simulink model "TV_2018_HIL"  (R2016a)
settings: Solver=FixedStepAuto  StartTime=0.0  StopTime=inf  FixedStep=0.001  RelTol=1e-3
PreLoadFcn:
  | TV_2017_parameters
values from neighbouring files (symbols this model uses):
  battery_voltage = single(530)    [HIL_parameters.m]    (also in HIL_parameters_2018.m; TV_2017_parameters.m; TV_2017_parameters_VD.m)
  car_params = Simulink_Car_params    [HIL_parameters.m]    (also in HIL_parameters_2018.m; TV_2017_parameters.m; TV_2017_parameters_VD.m)
  i_Diff = 16    [HIL_parameters.m]    (also in HIL_parameters_2018.m; TV_2017_parameters.m)
  Kp = 1    [HIL_parameters.m]    (also in HIL_parameters_2018.m; TV_2017_parameters.m; TV_2017_parameters_VD.m)
  motor_data = struct    [HIL_parameters.m]    (also in HIL_parameters_2018.m; TV_2017_parameters.m)
  powerLimitControl = Simulink_el    [HIL_parameters.m]    (also in HIL_parameters_2018.m; TV_2017_parameters.m; TV_2017_parameters_VD.m)
  settings = Simulink_Settings    [HIL_parameters.m]    (also in HIL_parameters_2018.m; TV_2017_parameters.m; TV_2017_parameters_VD.m)
  SpdC_BCC = 0    [HIL_parameters.m]    (also in HIL_parameters_2018.m; TV_2017_parameters.m; TV_2017_parameters_VD.m)
  Speed_Neg_sat = -21    [HIL_parameters.m]    (also in HIL_parameters_2018.m; TV_2017_parameters.m; TV_2017_parameters_VD.m)
  Speed_Pos_sat = 21    [HIL_parameters.m]    (also in HIL_parameters_2018.m; TV_2017_parameters.m; TV_2017_parameters_VD.m)
  SteeringAngleFL = [-23.80 -22.65 -21.50 -20.34 -19.18 -18.03 -16.86 -15.70 -14.53 -13.35 -12.18 -10.99 -9.80 -8.61 -7.40 -6.19 -4.97 -3.75 -2.51 -1.26 0 1.27 2.56 3.85 5.17 6.50 7.84 9.21 10.59 12.00 13.42 14.88 16.36 17.87 19.41 20.99 22.61 24.26 25.97 27.73 29.54]    [CarSetupAnalysis2018.m]    (also in HIL_parameters_2018.m; TV_2017_parameters.m; TV_2017_parameters_VD.m = [-24.129 -22.950 -21.772 -20.593 -19.413 -18.232 -17.050 -15)
  SteeringAngleFR = [-29.54 -27.73 -25.97 -24.26 -22.61 -20.99 -19.41 -17.87 -16.36 -14.88 -13.42 -12.00 -10.59 -9.21 -7.84 -6.50 -5.17 -3.85 -2.56 -1.27 0 1.26 2.51 3.75 4.97 6.19 7.40 8.61 9.80 10.99 12.18 13.35 14.53 15.70 16.86 18.03 19.18 20.34 21.50 22.65 23.80]    [CarSetupAnalysis2018.m]    (also in HIL_parameters_2018.m; TV_2017_parameters.m; TV_2017_parameters_VD.m = [-29.3050 -27.5340 -25.8140 -24.1410 -22.5110 -20.9180 -19.3)
  SteeringWhAngle = [-105 -99.75 -94.5 -89.25 -84 -78.75 -73.5 -68.25 -63 -57.75 -52.5 -47.25 -42 -36.75 -31.5 -26.25 -21.0 -15.75 -10.5 -5.25 0.0 5.25 10.50 15.75 21.00 26.25 31.50 36.75 42.00 47.25 52.50 57.75  63.00 68.25 73.50 78.75 84.00 89.25 94.50 99.75 105.00]    [TV_2017_parameters_VD.m]
  Tn_n = 0    [HIL_parameters.m]    (also in HIL_parameters_2018.m; TV_2017_parameters.m; TV_2017_parameters_VD.m)
  tractionControl = Simulink_tc    [HIL_parameters.m]    (also in HIL_parameters_2018.m; IterativeTractionControlTuning.m; TV_2017_parameters.m; TV_2017_parameters_VD.m)
  yawMomentGenerator = struct    [HIL_parameters.m]    (also in HIL_parameters_2018.m = Simulink_yawRate2; TV_2017_parameters.m = Simulink_yawRate2)
  yawRateControl = Simulink_yawRate    [HIL_parameters.m]    (also in HIL_parameters_2018.m; TV_2017_parameters.m; TV_2017_parameters_VD.m)
undefined symbols (not defined in the file or in its folder): canChannel, DiscIntNeverNeededParam, magnitude, speedEstimation, TC_Decr_Gas, TC_Derivative, TC_Incr_Gas, TC_On, TC_Relay_Off, TC_Relay_On
libraries: CarMaker4SL x366, simulink_extras x63, canmsglib x55, canlib x41, simulink x37, dspfdesign x2, sldrtlib x1
(part 3 of 15)

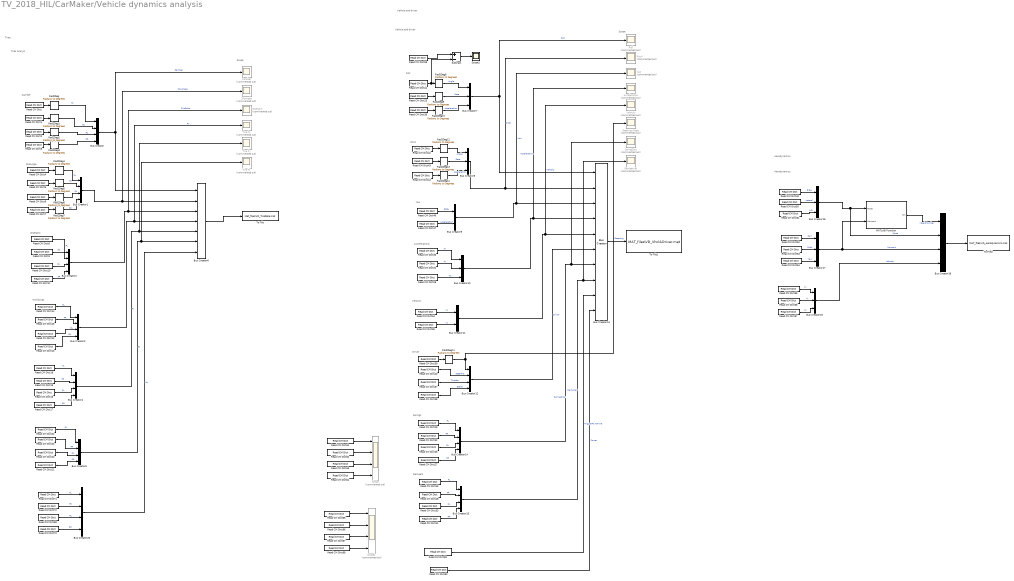
== system TV_2018_HIL/CarMaker/Vehicle dynamics analysis ==
  note: Aerodynamics
  note: Scope
  note: Scope
  note: Dampers
  note: Springs
  note: Driver
  note: Velocity
  note: Tire forces
  note: SlipRatio
  note: SlipAngle
  note: Camber
  note: Tires analyis
  note: Tires
  note: Accelerations
  note: Yaw
  note: Pitch
  note: Roll
  note: Vehicle and driver
  note: Vehicle and driver
  note: Aerodynamics
  Acceleration : Scope  Commented=on
  Bus Creator{,1..5,12,14..15,18,20} (11 alike) : BusCreator  Inputs=4
  Bus Creator{7..8,10,16..17,19} (6 alike) : BusCreator  Inputs=3
  Bus Creator11 : BusCreator  Inputs=2
  Bus Creator13 : BusCreator  Inputs=10
  Bus Creator6 : BusCreator  Inputs=7
  Bus Creator9 : BusCreator  Inputs=2
  Camber : Scope  Commented=on
  DamperVel : Scope  Commented=on
  MATLAB Function : MATLAB Function  TreatAsAtomicUnit=on
  Pitch : Scope  Commented=on
  Rad2Deg{,1..14} (15 alike) : simulink_extras/Transformations/Radians to Degrees
  Read CM Dict : CarMaker4SL/Read CM Dict  xname=Car.CamberFL  xsync=off
  Read CM Dict1 : CarMaker4SL/Read CM Dict  xname=Car.CamberFR  xsync=off
  Read CM Dict10 : CarMaker4SL/Read CM Dict  xname=Vhcl.RL.LongSlip  xsync=off
  Read CM Dict11 : CarMaker4SL/Read CM Dict  xname=Vhcl.RR.LongSlip  xsync=off
  Read CM Dict12 : CarMaker4SL/Read CM Dict  xname=Vhcl.RL.Fx  xsync=off
  Read CM Dict13 : CarMaker4SL/Read CM Dict  xname=Vhcl.RR.Fx  xsync=off
  Read CM Dict14 : CarMaker4SL/Read CM Dict  xname=Vhcl.FL.Fx  xsync=off
  Read CM Dict15 : CarMaker4SL/Read CM Dict  xname=Vhcl.FR.Fx  xsync=off
  Read CM Dict16 : CarMaker4SL/Read CM Dict  xname=Vhcl.RL.Fy  xsync=off
  Read CM Dict17 : CarMaker4SL/Read CM Dict  xname=Vhcl.RR.Fy  xsync=off
  Read CM Dict18 : CarMaker4SL/Read CM Dict  xname=Vhcl.FL.Fy  xsync=off
  Read CM Dict19 : CarMaker4SL/Read CM Dict  xname=Vhcl.FR.Fy  xsync=off
  Read CM Dict2 : CarMaker4SL/Read CM Dict  xname=Car.CamberRL  xsync=off
  Read CM Dict20 : CarMaker4SL/Read CM Dict  xname=Vhcl.RL.Fz  xsync=off
  Read CM Dict21 : CarMaker4SL/Read CM Dict  xname=Vhcl.RR.Fz  xsync=off
  Read CM Dict22 : CarMaker4SL/Read CM Dict  xname=Vhcl.FL.Fz  xsync=off
  Read CM Dict23 : CarMaker4SL/Read CM Dict  xname=Vhcl.FR.Fz  xsync=off
  Read CM Dict24 : CarMaker4SL/Read CM Dict  xname=Vhcl.Roll  xsync=off
  Read CM Dict25 : CarMaker4SL/Read CM Dict  xname=Vhcl.RollVel  xsync=off
  Read CM Dict26 : CarMaker4SL/Read CM Dict  xname=Car.SpringRL.l  xsync=off
  Read CM Dict27 : CarMaker4SL/Read CM Dict  xname=Car.SpringRR.l  xsync=off
  Read CM Dict28 : CarMaker4SL/Read CM Dict  xname=Car.az  xsync=off
  Read CM Dict29 : CarMaker4SL/Read CM Dict  xname=Car.SpringFL.l  xsync=off
  Read CM Dict3 : CarMaker4SL/Read CM Dict  xname=Car.CamberRR  xsync=off
  Read CM Dict30 : CarMaker4SL/Read CM Dict  xname=Car.ax  xsync=off
  Read CM Dict31 : CarMaker4SL/Read CM Dict  xname=Car.ay  xsync=off
  Read CM Dict32 : CarMaker4SL/Read CM Dict  xname=Car.SpringFR.l  xsync=off
  Read CM Dict33 : CarMaker4SL/Read CM Dict  xname=Car.DampRL.v  xsync=off
  Read CM Dict34 : CarMaker4SL/Read CM Dict  xname=Car.vx  xsync=off
  Read CM Dict35 : CarMaker4SL/Read CM Dict  xname=Car.vy  xsync=off
  Read CM Dict36 : CarMaker4SL/Read CM Dict  xname=Vhcl.RollAcc  xsync=off
  Read CM Dict37 : CarMaker4SL/Read CM Dict  xname=Driver.Gas  xsync=off
  Read CM Dict38 : CarMaker4SL/Read CM Dict  xname=Driver.Brake  xsync=off
  Read CM Dict39 : CarMaker4SL/Read CM Dict  xname=Vhcl.Steer.Ang  xsync=off
  Read CM Dict4 : CarMaker4SL/Read CM Dict  xname=Vhcl.FL.SideSlip  xsync=off
  Read CM Dict40 : CarMaker4SL/Read CM Dict  xname=Vhcl.Steer.Trq  xsync=off
  Read CM Dict41 : CarMaker4SL/Read CM Dict  xname=Car.DampRR.v  xsync=off
  Read CM Dict42 : CarMaker4SL/Read CM Dict  xname=Vhcl.Pitch  xsync=off
  Read CM Dict43 : CarMaker4SL/Read CM Dict  xname=Vhcl.PitchVel  xsync=off
  Read CM Dict44 : CarMaker4SL/Read CM Dict  xname=Vhcl.PitchAcc  xsync=off
  Read CM Dict45 : CarMaker4SL/Read CM Dict  xname=Car.DampFL.v  xsync=off
  Read CM Dict46 : CarMaker4SL/Read CM Dict  xname=Vhcl.YawRate  xsync=off
  Read CM Dict47 : CarMaker4SL/Read CM Dict  xname=Vhcl.YawAcc  xsync=off
  Read CM Dict48 : CarMaker4SL/Read CM Dict  xname=Car.DampFR.v  xsync=off
  Read CM Dict49 : CarMaker4SL/Read CM Dict  xname=Car.Aero.Frc_1.x  xsync=off
  Read CM Dict5 : CarMaker4SL/Read CM Dict  xname=Vhcl.FR.SideSlip  xsync=off
  Read CM Dict50 : CarMaker4SL/Read CM Dict  xname=Car.Aero.Frc_1.y  xsync=off
  Read CM Dict51 : CarMaker4SL/Read CM Dict  xname=Car.Aero.Frc_1.z  xsync=off
  Read CM Dict52 : CarMaker4SL/Read CM Dict  xname=Car.Aero.Trq_1.x  xsync=off
  Read CM Dict53 : CarMaker4SL/Read CM Dict  xname=Car.Aero.Trq_1.y  xsync=off
  Read CM Dict54 : CarMaker4SL/Read CM Dict  xname=Car.Aero.Trq_1.z  xsync=off
  Read CM Dict55 : CarMaker4SL/Read CM Dict  xname=Car.Aero.vres_1.x  xsync=off
  Read CM Dict56 : CarMaker4SL/Read CM Dict  xname=Car.Aero.vres_1.y  xsync=off
  Read CM Dict57 : CarMaker4SL/Read CM Dict  xname=Car.Aero.vres_1.z  xsync=off
  Read CM Dict58 : CarMaker4SL/Read CM Dict  xname=DM.TriggerPoint.Time  xsync=off
  Read CM Dict59 : CarMaker4SL/Read CM Dict  xname=Car.Roll  xsync=off
  Read CM Dict6 : CarMaker4SL/Read CM Dict  xname=Vhcl.RL.SideSlip  xsync=off
  Read CM Dict60 : CarMaker4SL/Read CM Dict  xname=Power  xsync=off
  Read CM Dict61 : CarMaker4SL/Read CM Dict  xname=Car.SpringFL.Frc_tot  xsync=off
  Read CM Dict62 : CarMaker4SL/Read CM Dict  xname=Car.SpringFR.Frc_tot  xsync=off
  Read CM Dict63 : CarMaker4SL/Read CM Dict  xname=Car.SpringRL.Frc_tot  xsync=off
  Read CM Dict64 : CarMaker4SL/Read CM Dict  xname=Car.SpringRR.Frc_tot  xsync=off
  Read CM Dict65 : CarMaker4SL/Read CM Dict  xname=Car.DampFL.Frc_tot  xsync=off
  Read CM Dict66 : CarMaker4SL/Read CM Dict  xname=Car.DampFR.Frc_tot  xsync=off
  Read CM Dict67 : CarMaker4SL/Read CM Dict  xname=Car.DampRL.Frc_tot  xsync=off
  Read CM Dict68 : CarMaker4SL/Read CM Dict  xname=Car.DampRR.Frc_tot  xsync=off
  Read CM Dict69 : CarMaker4SL/Read CM Dict  xname=Car.TrqAlignRL  xsync=off
  Read CM Dict7 : CarMaker4SL/Read CM Dict  xname=Vhcl.RR.SideSlip  xsync=off
  Read CM Dict70 : CarMaker4SL/Read CM Dict  xname=Car.TrqAlignRR  xsync=off
  Read CM Dict71 : CarMaker4SL/Read CM Dict  xname=Car.TrqAlignFL  xsync=off
  Read CM Dict72 : CarMaker4SL/Read CM Dict  xname=Car.TrqAlignFR  xsync=off
  Read CM Dict8 : CarMaker4SL/Read CM Dict  xname=Vhcl.FL.LongSlip  xsync=off
  Read CM Dict9 : CarMaker4SL/Read CM Dict  xname=Vhcl.FR.LongSlip  xsync=off
  Roll : Scope  Commented=on
  Scope : Scope  Commented=on  NumInputPorts=4
  Scope1 : Scope
  Scope2 : Scope  Commented=on  NumInputPorts=4
  SlipAngle : Scope  Commented=on
  SlipRatio : Scope  Commented=on
  SpringDisp : Scope  Commented=on
  Steering Angle : Scope  Commented=on
  Subtract : Sum  Inputs=+-
  Tire Fx : Scope  Commented=on
  Tire Fy : Scope  Commented=on
  Tire Fz : Scope  Commented=on
  To File : ToFile  Filename=Mat_files\VD_TireData.mat  MatrixName=Tire  SaveFormat=Timeseries
      settings: Decimation=2
  To File1 : ToFile  Filename=MAT_files\VD_Vhcl&Driver.mat  MatrixName=Vhcl  SaveFormat=Timeseries
      settings: Decimation=2
  To File2 : ToFile  Filename=MAT_files\VD_Aerodynamics.mat  MatrixName=Aero  SaveFormat=Timeseries
      settings: Decimation=2
  Velocity : Scope  Commented=on
  Yaw : Scope  Commented=on
  wires:
  Rad2Deg3/1 -> Bus Creator/4  "RR"
  Read CM Dict2/1 -> Rad2Deg2/1
  Rad2Deg/1 -> Bus Creator/1  "FL"
  Rad2Deg2/1 -> Bus Creator/3  "RL"
  Read CM Dict/1 -> Rad2Deg/1
  Rad2Deg1/1 -> Bus Creator/2  "FR"
  Read CM Dict1/1 -> Rad2Deg1/1
  Read CM Dict3/1 -> Rad2Deg3/1
  Rad2Deg7/1 -> Bus Creator1/4  "RR"
  Read CM Dict6/1 -> Rad2Deg6/1
  Rad2Deg4/1 -> Bus Creator1/1  "FL"
  Rad2Deg6/1 -> Bus Creator1/3  "RL"
  Read CM Dict4/1 -> Rad2Deg4/1
  Rad2Deg5/1 -> Bus Creator1/2  "FR"
  Read CM Dict5/1 -> Rad2Deg5/1
  Read CM Dict7/1 -> Rad2Deg7/1
  Read CM Dict11/1 -> Bus Creator2/4  "RR"
  Read CM Dict8/1 -> Bus Creator2/1  "FL"
  Read CM Dict10/1 -> Bus Creator2/3  "RL"
  Read CM Dict9/1 -> Bus Creator2/2  "FR"
  Read CM Dict13/1 -> Bus Creator3/4  "RR"
  Read CM Dict14/1 -> Bus Creator3/1  "FL"
  Read CM Dict12/1 -> Bus Creator3/3  "RL"
  Read CM Dict15/1 -> Bus Creator3/2  "FR"
  Read CM Dict17/1 -> Bus Creator4/4  "RR"
  Read CM Dict18/1 -> Bus Creator4/1  "FL"
  Read CM Dict16/1 -> Bus Creator4/3  "RL"
  Read CM Dict19/1 -> Bus Creator4/2  "FR"
  Read CM Dict21/1 -> Bus Creator5/4  "RR"
  Read CM Dict22/1 -> Bus Creator5/1  "FL"
  Read CM Dict20/1 -> Bus Creator5/3  "RL"
  Bus Creator/1 -> Bus Creator6/1, Camber/1  "Camber"
  Bus Creator1/1 -> SlipAngle/1, Bus Creator6/2  "SlipAngle"
  Bus Creator2/1 -> SlipRatio/1, Bus Creator6/3  "SlipRatio"
  Bus Creator3/1 -> Bus Creator6/4, Tire Fx/1  "Fx"
  Bus Creator4/1 -> Tire Fy/1, Bus Creator6/5  "Fy"
  Bus Creator5/1 -> Tire Fz/1, Bus Creator6/6  "Fz"
  Read CM Dict23/1 -> Bus Creator5/2  "FR"
  Bus Creator6/1 -> To File/1
  Read CM Dict36/1 -> Rad2Deg10/1
  Rad2Deg8/1 -> Bus Creator7/1  "Angle"
  Rad2Deg10/1 -> Bus Creator7/3  "Acceleration"
  Read CM Dict24/1 -> Subtract/2, Rad2Deg8/1
  Rad2Deg9/1 -> Bus Creator7/2  "Rate"
  Read CM Dict25/1 -> Rad2Deg9/1
  Read CM Dict44/1 -> Rad2Deg14/1
  Rad2Deg12/1 -> Bus Creator8/1  "Angle"
  Rad2Deg14/1 -> Bus Creator8/3  "Acceleration"
  Read CM Dict42/1 -> Rad2Deg12/1
  Rad2Deg13/1 -> Bus Creator8/2  "Rate"
  Read CM Dict43/1 -> Rad2Deg13/1
  Read CM Dict46/1 -> Bus Creator9/1  "Rate"
  Read CM Dict47/1 -> Bus Creator9/2  "Acceleration"
  Read CM Dict34/1 -> Bus Creator11/1  "Vx"
  Read CM Dict35/1 -> Bus Creator11/2  "Vy"
  Read CM Dict38/1 -> Bus Creator12/4  "Brake"
  Read CM Dict39/1 -> Rad2Deg11/1
  Read CM Dict37/1 -> Bus Creator12/3  "Throttle"
  Bus Creator7/1 -> Bus Creator13/1, Roll/1  "Roll"
  Bus Creator8/1 -> Pitch/1, Bus Creator13/2  "Pitch"
  Bus Creator9/1 -> Bus Creator13/3, Yaw/1  "Yaw"
  Bus Creator11/1 -> Velocity/1, Bus Creator13/5  "Velocity"
  Bus Creator12/1 -> Bus Creator13/6  "Driver"
  Read CM Dict40/1 -> Bus Creator12/2  "SteerTrq"
  Bus Creator13/1 -> To File1/1
  Rad2Deg11/1 -> Bus Creator12/1, Steering Angle/1  "SteerAng"
  Bus Creator10/1 -> Acceleration/1, Bus Creator13/4  "Acceleration"
  Read CM Dict27/1 -> Bus Creator14/4  "RR"
  Read CM Dict29/1 -> Bus Creator14/1  "FL"
  Read CM Dict26/1 -> Bus Creator14/3  "RL"
  Read CM Dict32/1 -> Bus Creator14/2  "FR"
  Bus Creator14/1 -> SpringDisp/1, Bus Creator13/7  "SpringDisp"
  Read CM Dict41/1 -> Bus Creator15/4  "RR"
  Read CM Dict45/1 -> Bus Creator15/1  "FL"
  Read CM Dict33/1 -> Bus Creator15/3  "RL"
  Read CM Dict48/1 -> Bus Creator15/2  "FR"
  Bus Creator15/1 -> DamperVel/1, Bus Creator13/8  "DampVel"
  Read CM Dict30/1 -> Bus Creator10/1  "Ax"
  Read CM Dict31/1 -> Bus Creator10/2  "Ay"
  Read CM Dict28/1 -> Bus Creator10/3  "Az"
  Read CM Dict49/1 -> Bus Creator16/1  "Drag"
  Read CM Dict50/1 -> Bus Creator16/2  "Lateral"
  Read CM Dict51/1 -> Bus Creator16/3  "Lift"
  Read CM Dict52/1 -> Bus Creator17/1  "Roll"
  Read CM Dict53/1 -> Bus Creator17/2  "Pitch"
  Read CM Dict54/1 -> Bus Creator17/3  "Yaw"
  Bus Creator16/1 -> Bus Creator18/2, MATLAB Function/1(Force)  "Force"
  Bus Creator17/1 -> MATLAB Function/2(Moment), Bus Creator18/3  "Moment"
  MATLAB Function/1(MM) -> Bus Creator18/1  "MagicMumber"
  Read CM Dict55/1 -> Bus Creator19/1  "Vx"
  Read CM Dict56/1 -> Bus Creator19/2  "Vy"
  Read CM Dict57/1 -> Bus Creator19/3  "Vz"
  Bus Creator19/1 -> Bus Creator18/4  "Velocity"
  Bus Creator18/1 -> To File2/1
  Read CM Dict59/1 -> Subtract/1
  Subtract/1 -> Scope1/1
  Read CM Dict60/1 -> Bus Creator13/10  "Power"
  Read CM Dict58/1 -> Bus Creator13/9  "TriggerPointTime"
  Read CM Dict61/1 -> Scope/1
  Read CM Dict62/1 -> Scope/2
  Read CM Dict63/1 -> Scope/3
  Read CM Dict64/1 -> Scope/4
  Read CM Dict65/1 -> Scope2/1
  Read CM Dict66/1 -> Scope2/2
  Read CM Dict67/1 -> Scope2/3
  Read CM Dict68/1 -> Scope2/4
  Read CM Dict70/1 -> Bus Creator20/4  "RR"
  Read CM Dict71/1 -> Bus Creator20/1  "FL"
  Read CM Dict69/1 -> Bus Creator20/3  "RL"
  Read CM Dict72/1 -> Bus Creator20/2  "FR"
  Bus Creator20/1 -> Bus Creator6/7  "Mz"

== system TV_2018_HIL/CarMaker/VehicleControl3 ==
  note: <Your model here>
  note: When implementing a vehicle control model,
      | be sure to add '-disablevehiclecontrol' to the command line arguments
      | in the CarMaker Model Configuration block.
      | Otherwise your model will possibly not see the original DrivMan signals
      | on its inputs, but those of a currently activated C-coded vehicle control model instead.
  Sync_In : Inport
  DrivMan.In : Inport  Port=2
  Bus Creator2 : BusCreator  Inputs=2
  CreateBus Vhcl.Misc : Subsystem
  CreateBus Vhcl.Wheel.In : Subsystem
  CreateBus VhclCtrl : Subsystem
  CreateBus VhclCtrl.PT : Subsystem
  CreateBus VhclCtrl.Steering : Subsystem
  Demux2 : Demux  Outputs=2
  VehicleControl : S-Function  FunctionName=CM_Sfun  Parameters='VehicleControl'  SFunctionDeploymentMode=off  EnableBusSupport=off
  VehicleControlUpd : S-Function  FunctionName=CM_Sfun  Parameters='VehicleControlUpd'  SFunctionDeploymentMode=off  EnableBusSupport=off
  Sync_Out : Outport
  Vhcl.Model.Source : Outport  Port=2
  VhclCtrl.Steering : Outport  Port=3
  Vhcl.Wheel.In : Outport  Port=4
  Vhcl.Misc : Outport  Port=5
  VhclCtrl.Brake : Outport  Port=6
  VhclCtrl.PT : Outport  Port=7
  wires:
  CreateBus VhclCtrl/1(Out) -> VehicleControlUpd/2
  VehicleControl/2 -> CreateBus VhclCtrl/1(In)
  VehicleControlUpd/2 -> Vhcl.Model.Source/1
  VehicleControlUpd/4 -> CreateBus Vhcl.Wheel.In/1(In1)
  VehicleControlUpd/5 -> CreateBus Vhcl.Misc/1(In1)
  VehicleControlUpd/6 -> Demux2/1
  VehicleControlUpd/7 -> CreateBus VhclCtrl.PT/1(In1)
  VehicleControlUpd/3 -> CreateBus VhclCtrl.Steering/1(In1)
  CreateBus Vhcl.Misc/1(Out1) -> Vhcl.Misc/1
  CreateBus Vhcl.Wheel.In/1(Out1) -> Vhcl.Wheel.In/1
  DrivMan.In/1 -> VehicleControl/2
  VehicleControl/1 -> VehicleControlUpd/1
  Sync_In/1 -> VehicleControl/1
  CreateBus VhclCtrl.PT/1(Out1) -> VhclCtrl.PT/1
  Bus Creator2/1 -> VhclCtrl.Brake/1
  CreateBus VhclCtrl.Steering/1(Out1) -> VhclCtrl.Steering/1
  VehicleControlUpd/1 -> Sync_Out/1
  Demux2/2 -> Bus Creator2/2  "VhclCtrl BrakePark"
  Demux2/1 -> Bus Creator2/1  "VhclCtrl Brake"

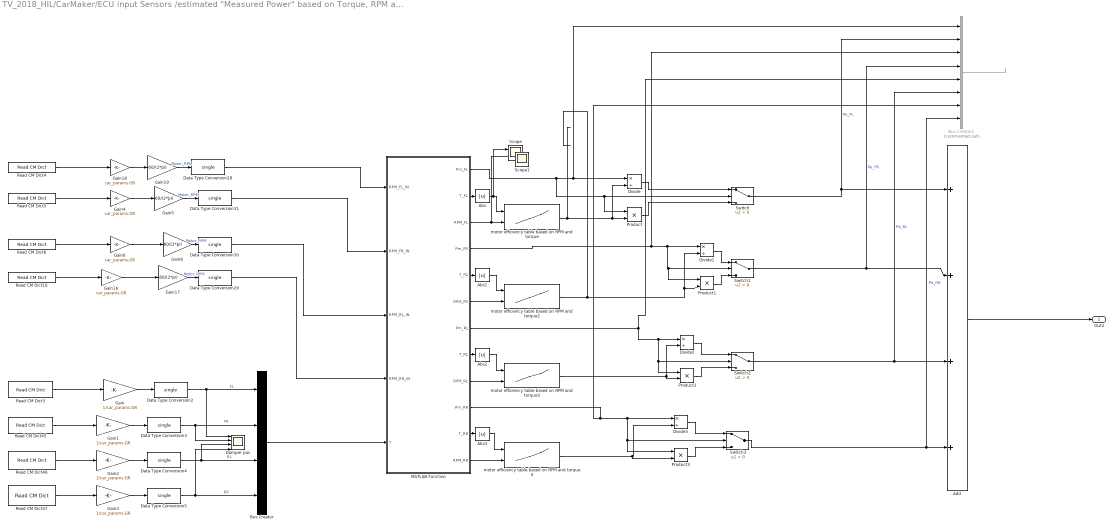
== system TV_2018_HIL/CarMaker/ECU input Sensors /estimated "Measured Power" based on Torque, RPM and datasheet IRL this is measured ==
  Abs{,1..3} (4 alike) : Abs
  Add : Sum  Inputs=++++
  Bus Creator : BusCreator  Inputs=4  OutDataTypeStr=Bus: T_meas
      settings: InheritFromInputs=off
  Bus Creator1 : BusCreator  Commented=on  Inputs=8  OutDataTypeStr=Bus: PowerDebug
      settings: InheritFromInputs=off
  Damper pos : Scope  NumInputPorts=4
  Data Type Conversion{2..5,28..31} (8 alike) : DataTypeConversion  OutDataTypeStr=single
  Divide{,1..3} (4 alike) : Product  Inputs=*/
  Gain{,1..3} (4 alike) : Gain  Gain=1/car_params.GR
  Gain{4,6,16,18} (4 alike) : Gain  Gain=car_params.GR
  Gain{5,8,17,19} (4 alike) : Gain  Gain=60/(2*pi)
  MATLAB Function : MATLAB Function  TreatAsAtomicUnit=on
  Product{,1..3} (4 alike) : Product
  Read CM Dict16 : CarMaker4SL/Read CM Dict  xname=Car.WheelSpd_RR  xsync=off
  Read CM Dict3 : CarMaker4SL/Read CM Dict  xname=PT.WFL.Trq_Drive  xsync=off
  Read CM Dict4 : CarMaker4SL/Read CM Dict  xname=Car.WheelSpd_FL  xsync=off
  Read CM Dict45 : CarMaker4SL/Read CM Dict  xname=PT.WFR.Trq_Drive  xsync=off
  Read CM Dict46 : CarMaker4SL/Read CM Dict  xname=PT.WRL.Trq_Drive  xsync=off
  Read CM Dict47 : CarMaker4SL/Read CM Dict  xname=PT.WRR.Trq_Drive  xsync=off
  Read CM Dict5 : CarMaker4SL/Read CM Dict  xname=Car.WheelSpd_FR  xsync=off
  Read CM Dict6 : CarMaker4SL/Read CM Dict  xname=Car.WheelSpd_RL  xsync=off
  Scope : Scope  NumInputPorts=2
  Scope1 : Scope  NumInputPorts=2
  Switch{,1..3} (4 alike) : Switch  Criteria=u2 > Threshold
  motor efficiency table based on RPM and torque : Lookup_n-D  BreakpointsForDimension1=single([1.3,2.7,5.4,7.9,10.4,12.5,14.4,16.0,17.4,18.5,19.6]);  BreakpointsForDimension2=single([500,1000,2000,3000,4000,6000,10000,12000,15000,19000]);  Table=single(reshape([0.6437000036239624,0.5799999833106995,0.44999998807907104,0.3499999940395355,0.28999999165534973,0.23999999463558197,0.20000000298023224,0.17000000178813934,0.14000000059604645,0.12999999523162842,0.10999999940395355,0.7099999785423279,0.699999988079071,0.6100000143051148,0.5099999904632568,0.4399999976158142,0.3799999952316284,0.33000001311302185,0.28999999165534973,0.25,0.2199999988079071,0.20000000298023224,0.7300000190734863,0.7699999809265137,0.7300000190734863,0.6700000166893005,0.6100000143051148,0.550000011920929,0.5,0.44999998807907104,0.4000000059604645,0.36000001430511475,0.33000001311302185,0.7400000095367432,0.800000011920929,0.7900000214576721,0.7400000095367432,0.6899999976158142,0.6399999856948853,0.5899999737739563,0.5400000214576721,0.5,0.46000000834465027,0.41999998688697815,0.75,0.8199999928474426,0.8199999928474426,0.7799999713897705,0.7400000095367432,0.699999988079071,0.6600000262260437,0.6100000143051148,0.5699999928474426,0.5299999713897705,0.49000000953674316,0.7599999904632568,0.8399999737739563,0.8500000238418579,0.8299999833106995,0.800000011920929,0.7699999809265137,0.7400000095367432,0.699999988079071,0.6600000262260437,0.6200000047683716,0.5899999737739563,0.7699999809265137,0.8500000238418579,0.8799999952316284,0.8700000047683716,0.8600000143051148,0.8399999737739563,0.8100000023841858,0.7799999713897705,0.7599999904632568,0.7200000286102295,0.699999988079071,0.7699999809265137,0.8500000238418579,0.8899999856948853,0.8799999952316284,0.8700000047683716,0.8500000238418579,0.8299999833106995,0.8100000023841858,0.7799999713897705,0.7599999904632568,0.7300000190734863,0.7699999809265137,0.8600000143051148,0.8999999761581421,0.8999999761581421,0.8899999856948853,0.8700000047683716,0.8500000238418579,0.8299999833106995,0.8100000023841858,0.7900000214576721,0.6700000166893005,0.7799999713897705,0.8600000143051148,0.8999999761581421,0.9100000262260437,0.8999999761581421,0.8899999856948853,0.8700000047683716,0.8600000143051148,0.8299999833106995,0.7699999809265137,0.699999988079071],11,10));  ExtrapMethod=Clip  UseLastTableValue=on  InternalRulePriority=Speed  RndMeth=Simplest  InputSameDT=on
  motor efficiency table based on RPM and torque 4 : Lookup_n-D  BreakpointsForDimension1=single([1.3,2.7,5.4,7.9,10.4,12.5,14.4,16.0,17.4,18.5,19.6]);  BreakpointsForDimension2=single([500,1000,2000,3000,4000,6000,10000,12000,15000,19000]);  Table=single(reshape([0.6437000036239624,0.5799999833106995,0.44999998807907104,0.3499999940395355,0.28999999165534973,0.23999999463558197,0.20000000298023224,0.17000000178813934,0.14000000059604645,0.12999999523162842,0.10999999940395355,0.7099999785423279,0.699999988079071,0.6100000143051148,0.5099999904632568,0.4399999976158142,0.3799999952316284,0.33000001311302185,0.28999999165534973,0.25,0.2199999988079071,0.20000000298023224,0.7300000190734863,0.7699999809265137,0.7300000190734863,0.6700000166893005,0.6100000143051148,0.550000011920929,0.5,0.44999998807907104,0.4000000059604645,0.36000001430511475,0.33000001311302185,0.7400000095367432,0.800000011920929,0.7900000214576721,0.7400000095367432,0.6899999976158142,0.6399999856948853,0.5899999737739563,0.5400000214576721,0.5,0.46000000834465027,0.41999998688697815,0.75,0.8199999928474426,0.8199999928474426,0.7799999713897705,0.7400000095367432,0.699999988079071,0.6600000262260437,0.6100000143051148,0.5699999928474426,0.5299999713897705,0.49000000953674316,0.7599999904632568,0.8399999737739563,0.8500000238418579,0.8299999833106995,0.800000011920929,0.7699999809265137,0.7400000095367432,0.699999988079071,0.6600000262260437,0.6200000047683716,0.5899999737739563,0.7699999809265137,0.8500000238418579,0.8799999952316284,0.8700000047683716,0.8600000143051148,0.8399999737739563,0.8100000023841858,0.7799999713897705,0.7599999904632568,0.7200000286102295,0.699999988079071,0.7699999809265137,0.8500000238418579,0.8899999856948853,0.8799999952316284,0.8700000047683716,0.8500000238418579,0.8299999833106995,0.8100000023841858,0.7799999713897705,0.7599999904632568,0.7300000190734863,0.7699999809265137,0.8600000143051148,0.8999999761581421,0.8999999761581421,0.8899999856948853,0.8700000047683716,0.8500000238418579,0.8299999833106995,0.8100000023841858,0.7900000214576721,0.6700000166893005,0.7799999713897705,0.8600000143051148,0.8999999761581421,0.9100000262260437,0.8999999761581421,0.8899999856948853,0.8700000047683716,0.8600000143051148,0.8299999833106995,0.7699999809265137,0.699999988079071],11,10));  ExtrapMethod=Clip  UseLastTableValue=on  InternalRulePriority=Speed  RndMeth=Simplest  InputSameDT=on
  motor efficiency table based on RPM and torque2 : Lookup_n-D  BreakpointsForDimension1=single([1.3,2.7,5.4,7.9,10.4,12.5,14.4,16.0,17.4,18.5,19.6]);  BreakpointsForDimension2=single([500,1000,2000,3000,4000,6000,10000,12000,15000,19000]);  Table=single(reshape([0.6437000036239624,0.5799999833106995,0.44999998807907104,0.3499999940395355,0.28999999165534973,0.23999999463558197,0.20000000298023224,0.17000000178813934,0.14000000059604645,0.12999999523162842,0.10999999940395355,0.7099999785423279,0.699999988079071,0.6100000143051148,0.5099999904632568,0.4399999976158142,0.3799999952316284,0.33000001311302185,0.28999999165534973,0.25,0.2199999988079071,0.20000000298023224,0.7300000190734863,0.7699999809265137,0.7300000190734863,0.6700000166893005,0.6100000143051148,0.550000011920929,0.5,0.44999998807907104,0.4000000059604645,0.36000001430511475,0.33000001311302185,0.7400000095367432,0.800000011920929,0.7900000214576721,0.7400000095367432,0.6899999976158142,0.6399999856948853,0.5899999737739563,0.5400000214576721,0.5,0.46000000834465027,0.41999998688697815,0.75,0.8199999928474426,0.8199999928474426,0.7799999713897705,0.7400000095367432,0.699999988079071,0.6600000262260437,0.6100000143051148,0.5699999928474426,0.5299999713897705,0.49000000953674316,0.7599999904632568,0.8399999737739563,0.8500000238418579,0.8299999833106995,0.800000011920929,0.7699999809265137,0.7400000095367432,0.699999988079071,0.6600000262260437,0.6200000047683716,0.5899999737739563,0.7699999809265137,0.8500000238418579,0.8799999952316284,0.8700000047683716,0.8600000143051148,0.8399999737739563,0.8100000023841858,0.7799999713897705,0.7599999904632568,0.7200000286102295,0.699999988079071,0.7699999809265137,0.8500000238418579,0.8899999856948853,0.8799999952316284,0.8700000047683716,0.8500000238418579,0.8299999833106995,0.8100000023841858,0.7799999713897705,0.7599999904632568,0.7300000190734863,0.7699999809265137,0.8600000143051148,0.8999999761581421,0.8999999761581421,0.8899999856948853,0.8700000047683716,0.8500000238418579,0.8299999833106995,0.8100000023841858,0.7900000214576721,0.6700000166893005,0.7799999713897705,0.8600000143051148,0.8999999761581421,0.9100000262260437,0.8999999761581421,0.8899999856948853,0.8700000047683716,0.8600000143051148,0.8299999833106995,0.7699999809265137,0.699999988079071],11,10));  ExtrapMethod=Clip  UseLastTableValue=on  InternalRulePriority=Speed  RndMeth=Simplest  InputSameDT=on
  motor efficiency table based on RPM and torque3 : Lookup_n-D  BreakpointsForDimension1=single([1.3,2.7,5.4,7.9,10.4,12.5,14.4,16.0,17.4,18.5,19.6]);  BreakpointsForDimension2=single([500,1000,2000,3000,4000,6000,10000,12000,15000,19000]);  Table=single(reshape([0.6437000036239624,0.5799999833106995,0.44999998807907104,0.3499999940395355,0.28999999165534973,0.23999999463558197,0.20000000298023224,0.17000000178813934,0.14000000059604645,0.12999999523162842,0.10999999940395355,0.7099999785423279,0.699999988079071,0.6100000143051148,0.5099999904632568,0.4399999976158142,0.3799999952316284,0.33000001311302185,0.28999999165534973,0.25,0.2199999988079071,0.20000000298023224,0.7300000190734863,0.7699999809265137,0.7300000190734863,0.6700000166893005,0.6100000143051148,0.550000011920929,0.5,0.44999998807907104,0.4000000059604645,0.36000001430511475,0.33000001311302185,0.7400000095367432,0.800000011920929,0.7900000214576721,0.7400000095367432,0.6899999976158142,0.6399999856948853,0.5899999737739563,0.5400000214576721,0.5,0.46000000834465027,0.41999998688697815,0.75,0.8199999928474426,0.8199999928474426,0.7799999713897705,0.7400000095367432,0.699999988079071,0.6600000262260437,0.6100000143051148,0.5699999928474426,0.5299999713897705,0.49000000953674316,0.7599999904632568,0.8399999737739563,0.8500000238418579,0.8299999833106995,0.800000011920929,0.7699999809265137,0.7400000095367432,0.699999988079071,0.6600000262260437,0.6200000047683716,0.5899999737739563,0.7699999809265137,0.8500000238418579,0.8799999952316284,0.8700000047683716,0.8600000143051148,0.8399999737739563,0.8100000023841858,0.7799999713897705,0.7599999904632568,0.7200000286102295,0.699999988079071,0.7699999809265137,0.8500000238418579,0.8899999856948853,0.8799999952316284,0.8700000047683716,0.8500000238418579,0.8299999833106995,0.8100000023841858,0.7799999713897705,0.7599999904632568,0.7300000190734863,0.7699999809265137,0.8600000143051148,0.8999999761581421,0.8999999761581421,0.8899999856948853,0.8700000047683716,0.8500000238418579,0.8299999833106995,0.8100000023841858,0.7900000214576721,0.6700000166893005,0.7799999713897705,0.8600000143051148,0.8999999761581421,0.9100000262260437,0.8999999761581421,0.8899999856948853,0.8700000047683716,0.8600000143051148,0.8299999833106995,0.7699999809265137,0.699999988079071],11,10));  ExtrapMethod=Clip  UseLastTableValue=on  InternalRulePriority=Speed  RndMeth=Simplest  InputSameDT=on
  Out2 : Outport
  wires:
  MATLAB Function/3(RPM_FL) -> Scope1/1, motor efficiency table based on RPM and torque/2
  Data Type Conversion28/1 -> MATLAB Function/1(RPM_FL_IN)
  MATLAB Function/2(T_FL) -> Abs/1
  motor efficiency table based on RPM and torque 4/1 -> Product3/2, Divide3/2
  Divide1/1 -> Switch1/1
  Product1/1 -> Switch1/3
  MATLAB Function/10(Pm_RR) -> Switch3/2, Product3/1, Divide3/1, Bus Creator1/7
  motor efficiency table based on RPM and torque3/1 -> Product2/2, Divide2/2
  MATLAB Function/8(T_RL) -> Abs2/1
  Abs3/1 -> motor efficiency table based on RPM and torque 4/1
  Abs1/1 -> motor efficiency table based on RPM and torque2/1
  Bus Creator/1 -> MATLAB Function/5(T)
  MATLAB Function/12(RPM_RR) -> motor efficiency table based on RPM and torque 4/2
  MATLAB Function/1(Pm_FL) -> Product/1, Switch/2, Divide/1, Bus Creator1/1
  MATLAB Function/7(Pm_RL) -> Switch2/2, Product2/1, Divide2/1, Bus Creator1/5
  MATLAB Function/5(T_FR) -> Abs1/1
  MATLAB Function/11(T_RR) -> Abs3/1
  Data Type Conversion31/1 -> MATLAB Function/2(RPM_FR_IN)
  MATLAB Function/9(RPM_RL) -> motor efficiency table based on RPM and torque3/2
  Data Type Conversion30/1 -> MATLAB Function/3(RPM_RL_IN)
  Data Type Conversion29/1 -> MATLAB Function/4(RPM_RR_IN)
  Divide/1 -> Switch/1
  Product/1 -> Switch/3
  Abs2/1 -> motor efficiency table based on RPM and torque3/1
  motor efficiency table based on RPM and torque/1 -> Divide/2, Product/2
  MATLAB Function/4(Pm_FR) -> Bus Creator1/3, Product1/1, Switch1/2, Divide1/1
  Abs/1 -> Scope/1, motor efficiency table based on RPM and torque/1
  motor efficiency table based on RPM and torque2/1 -> Divide1/2, Product1/2
  MATLAB Function/6(RPM_FR) -> motor efficiency table based on RPM and torque2/2
  Switch/1 -> Bus Creator1/2, Add/1  "Pe_FL"
  Divide2/1 -> Switch2/1
  Product3/1 -> Switch3/3
  Switch2/1 -> Bus Creator1/6, Add/3  "Pe_RL"
  Product2/1 -> Switch2/3
  Switch1/1 -> Bus Creator1/4, Add/2  "Pe_FR"
  Switch3/1 -> Add/4, Bus Creator1/8  "Pe_RR"
  Divide3/1 -> Switch3/1
  Read CM Dict46/1 -> Gain2/1
  Read CM Dict3/1 -> Gain/1
  Read CM Dict45/1 -> Gain1/1
  Gain6/1 -> Gain8/1
  Data Type Conversion2/1 -> Damper pos/1, Bus Creator/1  "FL"
  Gain2/1 -> Data Type Conversion4/1
  Read CM Dict4/1 -> Gain18/1
  Read CM Dict6/1 -> Gain6/1
  Gain17/1 -> Data Type Conversion29/1  "Motor_RPM"
  Data Type Conversion5/1 -> Damper pos/4, Bus Creator/4  "RR"
  Gain/1 -> Data Type Conversion2/1
  Gain3/1 -> Data Type Conversion5/1
  Gain4/1 -> Gain5/1
  Read CM Dict47/1 -> Gain3/1
  Gain1/1 -> Data Type Conversion3/1
  Gain5/1 -> Data Type Conversion31/1  "Motor_RPM"
  Gain8/1 -> Data Type Conversion30/1  "Motor_RPM"
  Data Type Conversion4/1 -> Damper pos/3, Bus Creator/3  "RL"
  Data Type Conversion3/1 -> Damper pos/2, Bus Creator/2  "FR"
  Gain18/1 -> Gain19/1
  Read CM Dict16/1 -> Gain16/1
  Add/1 -> Out2/1
  Read CM Dict5/1 -> Gain4/1
  Gain16/1 -> Gain17/1
  Gain19/1 -> Data Type Conversion28/1  "Motor_RPM"
  Bus Creator1/1 -> ?

== system TV_2018_HIL/CarMaker/Function-Call Subsystem4/AMK Inverter Setpoints from ECU ==
  In1 : Inport
  In2 : Inport  Port=2
  In3 : Inport  Port=3
  In4 : Inport  Port=4
  In5 : Inport  Port=5
  In6 : Inport  Port=6
  CAN unpack AMK SETPOINTS_1    1 : canmsglib/CAN Unpack  MsgList=(none)  MsgName=ECU_SET_POINT_FL_ID  MsgIDType=Standard (11-bit identifier)  MsgIdentifier=ECU_SET_POINT_FL_ID  MsgLength=8  SignalInfo=AMK_Control$8$8$1$1$1$0$1$0$-Inf$Inf$#AMK_TargetVelocity_RPM$16$16$1$1$1$0$1$0$-Inf$Inf$#AMK_pos_lim$32$16$1$1$1$0$1$0$-Inf$Inf$#AMK_neg_lim$48$16$1$1$1$0$1$0$-Inf$Inf$#  NSignals=4  IDPort=off  TimestampPort=on  ErrorPort=off  RemotePort=off  LengthPort=off  StatusPort=off  StartBits=str2num('[int32(8);int32(16);int32(32);int32(48)]')  SignalSizes=str2num('[int32(8);int32(16);int32(16);int32(16)]')  ByteOrders=str2num('[int32(1);int32(1);int32(1);int32(1)]')  DataTypes=str2num('[int32(1);int32(1);int32(1);int32(1)]')  MultiplexTypes=str2num('[int32(1);int32(1);int32(1);int32(1)]')  MultiplexValues=str2num('[double(0);double(0);double(0);double(0)]')  Factors=str2num('[double(1);double(1);double(1);double(1)]')  Offsets=str2num('[double(0);double(0);double(0);double(0)]')  Minimums=str2num('[double(-Inf);double(-Inf);double(-Inf);double(-Inf)]')  Maximums=str2num('[double(Inf);double(Inf);double(Inf);double(Inf)]')
  CAN unpack AMK SETPOINTS_1    2 : canmsglib/CAN Unpack  MsgList=(none)  MsgName=ECU_SET_POINT_FR_ID  MsgIDType=Standard (11-bit identifier)  MsgIdentifier=ECU_SET_POINT_FR_ID  MsgLength=8  SignalInfo=AMK_Control$8$8$1$1$1$0$1$0$-Inf$Inf$#AMK_TargetVelocity_RPM$16$16$1$1$1$0$1$0$-Inf$Inf$#AMK_pos_lim$32$16$1$1$1$0$1$0$-Inf$Inf$#AMK_neg_lim$48$16$1$1$1$0$1$0$-Inf$Inf$#  NSignals=4  IDPort=off  TimestampPort=on  ErrorPort=off  RemotePort=off  LengthPort=off  StatusPort=off  StartBits=str2num('[int32(8);int32(16);int32(32);int32(48)]')  SignalSizes=str2num('[int32(8);int32(16);int32(16);int32(16)]')  ByteOrders=str2num('[int32(1);int32(1);int32(1);int32(1)]')  DataTypes=str2num('[int32(1);int32(1);int32(1);int32(1)]')  MultiplexTypes=str2num('[int32(1);int32(1);int32(1);int32(1)]')  MultiplexValues=str2num('[double(0);double(0);double(0);double(0)]')  Factors=str2num('[double(1);double(1);double(1);double(1)]')  Offsets=str2num('[double(0);double(0);double(0);double(0)]')  Minimums=str2num('[double(-Inf);double(-Inf);double(-Inf);double(-Inf)]')  Maximums=str2num('[double(Inf);double(Inf);double(Inf);double(Inf)]')
  CAN unpack AMK SETPOINTS_1    3 : canmsglib/CAN Unpack  MsgList=(none)  MsgName=ECU_SET_POINT_RL_ID  MsgIDType=Standard (11-bit identifier)  MsgIdentifier=ECU_SET_POINT_RL_ID  MsgLength=8  SignalInfo=AMK_Control$8$8$1$1$1$0$1$0$-Inf$Inf$#AMK_TargetVelocity_RPM$16$16$1$1$1$0$1$0$-Inf$Inf$#AMK_pos_lim$32$16$1$1$1$0$1$0$-Inf$Inf$#AMK_neg_lim$48$16$1$1$1$0$1$0$-Inf$Inf$#  NSignals=4  IDPort=off  TimestampPort=on  ErrorPort=off  RemotePort=off  LengthPort=off  StatusPort=off  StartBits=str2num('[int32(8);int32(16);int32(32);int32(48)]')  SignalSizes=str2num('[int32(8);int32(16);int32(16);int32(16)]')  ByteOrders=str2num('[int32(1);int32(1);int32(1);int32(1)]')  DataTypes=str2num('[int32(1);int32(1);int32(1);int32(1)]')  MultiplexTypes=str2num('[int32(1);int32(1);int32(1);int32(1)]')  MultiplexValues=str2num('[double(0);double(0);double(0);double(0)]')  Factors=str2num('[double(1);double(1);double(1);double(1)]')  Offsets=str2num('[double(0);double(0);double(0);double(0)]')  Minimums=str2num('[double(-Inf);double(-Inf);double(-Inf);double(-Inf)]')  Maximums=str2num('[double(Inf);double(Inf);double(Inf);double(Inf)]')
  CAN unpack AMK SETPOINTS_1    4 : canmsglib/CAN Unpack  MsgList=(none)  MsgName=ECU_SET_POINT_RR_ID  MsgIDType=Standard (11-bit identifier)  MsgIdentifier=ECU_SET_POINT_RR_ID  MsgLength=8  SignalInfo=AMK_Control$8$8$1$1$1$0$1$0$-Inf$Inf$#AMK_TargetVelocity_RPM$16$16$1$1$1$0$1$0$-Inf$Inf$#AMK_pos_lim$32$16$1$1$1$0$1$0$-Inf$Inf$#AMK_neg_lim$48$16$1$1$1$0$1$0$-Inf$Inf$#  NSignals=4  IDPort=off  TimestampPort=on  ErrorPort=off  RemotePort=off  LengthPort=off  StatusPort=off  StartBits=str2num('[int32(8);int32(16);int32(32);int32(48)]')  SignalSizes=str2num('[int32(8);int32(16);int32(16);int32(16)]')  ByteOrders=str2num('[int32(1);int32(1);int32(1);int32(1)]')  DataTypes=str2num('[int32(1);int32(1);int32(1);int32(1)]')  MultiplexTypes=str2num('[int32(1);int32(1);int32(1);int32(1)]')  MultiplexValues=str2num('[double(0);double(0);double(0);double(0)]')  Factors=str2num('[double(1);double(1);double(1);double(1)]')  Offsets=str2num('[double(0);double(0);double(0);double(0)]')  Minimums=str2num('[double(-Inf);double(-Inf);double(-Inf);double(-Inf)]')  Maximums=str2num('[double(Inf);double(Inf);double(Inf);double(Inf)]')
  Gain5 : Gain  Commented=through  Gain=0.001/3
  Gain6 : Gain  Commented=through  Gain=0.001/3
  MATLAB Function : MATLAB Function  Commented=through  TreatAsAtomicUnit=on
  MATLAB Function1 : MATLAB Function  Commented=through  TreatAsAtomicUnit=on
  MATLAB Function2 : MATLAB Function  Commented=through  TreatAsAtomicUnit=on
  MATLAB Function3 : MATLAB Function  Commented=through  TreatAsAtomicUnit=on
  Math Function1 : Math  Commented=through  Operator=reciprocal  RndMeth=Zero  SaturateOnIntegerOverflow=on
  Product : Product
  Scope1 : Scope  NumInputPorts=3
  Scope2 : Scope  NumInputPorts=3
  Scope3 : Scope  NumInputPorts=3
  Write CM Dict1 : CarMaker4SL/Write CM Dict  xname=Tlim_pos_FL  xsync=off
  Write CM Dict11 : CarMaker4SL/Write CM Dict  xname=Tlim_neg_FR  xsync=off
  Write CM Dict13 : CarMaker4SL/Write CM Dict  xname=w_set_FR  xsync=off
  Write CM Dict15 : CarMaker4SL/Write CM Dict  xname=Tlim_neg_RL  xsync=off
  Write CM Dict16 : CarMaker4SL/Write CM Dict  xname=w_set_RL  xsync=off
  Write CM Dict18 : CarMaker4SL/Write CM Dict  xname=Tlim_neg_RR  xsync=off
  Write CM Dict19 : CarMaker4SL/Write CM Dict  xname=w_set_RR  xsync=off
  Write CM Dict2 : CarMaker4SL/Write CM Dict  xname=Tlim_pos_FR  xsync=off
  Write CM Dict20 : CarMaker4SL/Write CM Dict  xname=Tlim_neg_FL  xsync=off
  Write CM Dict27 : CarMaker4SL/Write CM Dict  xname=w_set_FL  xsync=off
  Write CM Dict3 : CarMaker4SL/Write CM Dict  xname=Tlim_pos_RL  xsync=off
  Write CM Dict4 : CarMaker4SL/Write CM Dict  xname=Tlim_pos_RR  xsync=off
  Out1 : Outport
  Out2 : Outport  Port=2
  Out3 : Outport  Port=3
  Out4 : Outport  Port=4
  Out5 : Outport  Port=5
  Out6 : Outport  Port=6
  Out7 : Outport  Port=7
  Out8 : Outport  Port=8
  wires:
  CAN unpack AMK SETPOINTS_1    2/2 -> MATLAB Function1/1(w_set_16)
  CAN unpack AMK SETPOINTS_1    3/2 -> MATLAB Function2/1(w_set_16)
  MATLAB Function3/2(trq_pos_f) -> Write CM Dict4/1
  CAN unpack AMK SETPOINTS_1    3/5 -> Out6/1
  MATLAB Function1/2(trq_pos_f) -> Product/1, Write CM Dict2/1
  CAN unpack AMK SETPOINTS_1    4/5 -> Out8/1
  CAN unpack AMK SETPOINTS_1    2/3 -> MATLAB Function1/2(trq_pos_16)
  MATLAB Function3/3(trq_neg_f) -> Write CM Dict18/1
  CAN unpack AMK SETPOINTS_1    4/1 -> Out7/1
  CAN unpack AMK SETPOINTS_1    1/5 -> Out2/1
  CAN unpack AMK SETPOINTS_1    1/1 -> Out1/1
  CAN unpack AMK SETPOINTS_1    3/3 -> MATLAB Function2/2(trq_pos_16)
  MATLAB Function/2(trq_pos_f) -> Scope1/2, Write CM Dict1/1
  MATLAB Function1/1(w_set_f) -> Write CM Dict13/1
  Gain5/1 -> Scope1/1
  CAN unpack AMK SETPOINTS_1    4/4 -> MATLAB Function3/3(trq_neg_16)
  CAN unpack AMK SETPOINTS_1    3/4 -> MATLAB Function2/3(trq_neg_16)
  CAN unpack AMK SETPOINTS_1    2/1 -> Out3/1
  CAN unpack AMK SETPOINTS_1    4/3 -> MATLAB Function3/2(trq_pos_16)
  MATLAB Function1/3(trq_neg_f) -> Write CM Dict11/1
  CAN unpack AMK SETPOINTS_1    2/5 -> Out4/1
  CAN unpack AMK SETPOINTS_1    1/4 -> Scope3/3, MATLAB Function/3(trq_neg_16)  "t_FL"
  MATLAB Function2/1(w_set_f) -> Write CM Dict16/1
  Product/1 -> Scope2/2
  CAN unpack AMK SETPOINTS_1    4/2 -> MATLAB Function3/1(w_set_16)
  MATLAB Function2/3(trq_neg_f) -> Write CM Dict15/1
  CAN unpack AMK SETPOINTS_1    2/4 -> MATLAB Function1/3(trq_neg_16)
  MATLAB Function3/1(w_set_f) -> Write CM Dict19/1
  CAN unpack AMK SETPOINTS_1    3/1 -> Out5/1
  MATLAB Function2/2(trq_pos_f) -> Math Function1/1, Write CM Dict3/1
  MATLAB Function/3(trq_neg_f) -> Scope1/3, Write CM Dict20/1
  MATLAB Function/1(w_set_f) -> Write CM Dict27/1, Gain5/1
  Gain6/1 -> Scope3/1
  Math Function1/1 -> Product/2
  CAN unpack AMK SETPOINTS_1    1/2 -> Gain6/1, MATLAB Function/1(w_set_16)
  CAN unpack AMK SETPOINTS_1    1/3 -> Scope3/2, MATLAB Function/2(trq_pos_16)
  In6/1 -> CAN unpack AMK SETPOINTS_1    4/1
  In4/1 -> Scope2/3
  In1/1 -> CAN unpack AMK SETPOINTS_1    1/1
  In5/1 -> CAN unpack AMK SETPOINTS_1    3/1
  In3/1 -> Scope2/1
  In2/1 -> CAN unpack AMK SETPOINTS_1    2/1

== system TV_2018_HIL/CarMaker/IPG Vehicle3/Brake ==
  note: When replacing the entire braking system,
      | be sure to add '-disablebrake' to the command line arguments
      | in the CarMaker Model Configuration block.
  note: <Your model here>
  Sync_In : Inport
  Brake.IF.In : Inport  Port=2
  VhclCtrl.Brake : Inport  Port=3
  Brake : S-Function  FunctionName=CM_Sfun  Parameters='Brake'  SFunctionDeploymentMode=off  EnableBusSupport=off
  BrakeUpd : S-Function  FunctionName=CM_Sfun  Parameters='BrakeUpd'  SFunctionDeploymentMode=off  EnableBusSupport=off
  BusCreator1 : BusCreator  Inputs=16
  CreateBus Vhcl.Wheel.PT : Subsystem
  Demux : Demux  Outputs=16
  Sync_Out : Outport
  Vhcl.Wheel.PT : Outport  Port=2
  wires:
  Demux/16 -> BusCreator1/16  "Brake IF Trq_DriveSrc_trg d3"
  Demux/15 -> BusCreator1/15  "Brake IF Trq_DriveSrc_trg d2"
  Demux/14 -> BusCreator1/14  "Brake IF Trq_DriveSrc_trg d1"
  Demux/13 -> BusCreator1/13  "Brake IF Trq_DriveSrc_trg d0"
  Demux/12 -> BusCreator1/12  "Brake IF Trq_Reg_trg RR"
  Demux/11 -> BusCreator1/11  "Brake IF Trq_Reg_trg RL"
  Demux/10 -> BusCreator1/10  "Brake IF Trq_Reg_trg FR"
  Demux/9 -> BusCreator1/9  "Brake IF Trq_Reg_trg FL"
  Demux/8 -> BusCreator1/8  "Brake IF Trq_PB RR"
  Demux/7 -> BusCreator1/7  "Brake IF Trq_PB RL"
  Demux/6 -> BusCreator1/6  "Brake IF Trq_PB FR"
  Demux/5 -> BusCreator1/5  "Brake IF Trq_PB FL"
  Demux/4 -> BusCreator1/4  "Brake IF Trq_WB RR"
  Demux/3 -> BusCreator1/3  "Brake IF Trq_WB RL"
  Demux/2 -> BusCreator1/2  "Brake IF Trq_WB FR"
  Demux/1 -> BusCreator1/1  "Brake IF Trq_WB FL"
  Brake/2 -> Demux/1
  BusCreator1/1 -> BrakeUpd/2
  BrakeUpd/1 -> Sync_Out/1
  Brake/1 -> BrakeUpd/1  "Sync"
  Brake.IF.In/1 -> Brake/2
  VhclCtrl.Brake/1 -> Brake/3
  Sync_In/1 -> Brake/1
  BrakeUpd/2 -> CreateBus Vhcl.Wheel.PT/1(In)
  CreateBus Vhcl.Wheel.PT/1(Out) -> Vhcl.Wheel.PT/1

== system TV_2018_HIL/CarMaker/IPG Vehicle3/CarAndTrailer ==
  Sync_In : Inport
  VhclCtrl.Steering : Inport  Port=2
  Vhcl.Wheel.In : Inport  Port=3
  Vhcl.Misc : Inport  Port=4
  CarAndTrailerUpd : Subsystem
  Forces : Subsystem
  Ground : Ground
  Kinematics : Subsystem
  Kinetics : Subsystem
  Steering : Subsystem
  Terminator : Terminator
  Terminator1 : Terminator
  Trailer : Subsystem
  Sync_Out : Outport
  Brake.IF.In : Outport  Port=2
  wires:
  Trailer/9(Car.Hitch.FrcTrq) -> CarAndTrailerUpd/9(Car.Hitch.FrcTrq)
  Trailer/8(Vhcl.Wheel.RR) -> CarAndTrailerUpd/8(Vhcl.Wheel.RR)
  Trailer/7(Vhcl.Wheel.RL) -> CarAndTrailerUpd/7(Vhcl.Wheel.RL)
  Trailer/6(Vhcl.Wheel.FR) -> CarAndTrailerUpd/6(Vhcl.Wheel.FR)
  Trailer/5(Vhcl.Wheel.FL) -> CarAndTrailerUpd/5(Vhcl.Wheel.FL)
  Trailer/4(Vhcl.PoI) -> CarAndTrailerUpd/4(Vhcl.PoI)
  Trailer/3(Vhcl.Motion) -> CarAndTrailerUpd/3(Vhcl.Motion)
  Trailer/2(Vhcl.Steering) -> CarAndTrailerUpd/2(Vhcl.Steering)
  Trailer/1(Sync_Out) -> CarAndTrailerUpd/1(Sync_In)
  CarAndTrailerUpd/2(Brake.IF.In) -> Brake.IF.In/1
  CarAndTrailerUpd/1(Sync_Out) -> Sync_Out/1
  Vhcl.Misc/1 -> Terminator1/1
  Vhcl.Wheel.In/1 -> Terminator/1
  Kinetics/6(WheelCarrier.Misc) -> Trailer/6(WheelCarrier.Misc)
  Kinetics/5(Car.Trq_T2W) -> Trailer/5(Car.Trq_T2W)
  Steering/2(Steer.IF) -> Kinematics/2(Steer.IF)
  Kinetics/4(Car.Fr1) -> Trailer/4(Car.Fr1)
  Kinetics/3(Car.Hitch) -> Trailer/3(Car.Hitch)
  Kinetics/2(Trailer.Load) -> Trailer/2(Trailer.Load)
  VhclCtrl.Steering/1 -> Steering/2(VhclCtrl.Steering)
  Sync_In/1 -> Steering/1(Sync_In)
  Steering/1(Sync_Out) -> Kinematics/1(Sync_In)
  Kinetics/1(Sync_Out) -> Trailer/1(Sync_In)
  Ground/1 -> CarAndTrailerUpd/10(Vhcl.Fr1A)
  Forces/11(FStabi) -> Kinetics/11(FStabi)
  Forces/10(FDamp) -> Kinetics/10(FDamp)
  Forces/9(FSpring) -> Kinetics/9(FSpring)
  Forces/8(TireRR_Out) -> Kinetics/8(TireRR.Out)
  Forces/7(TireRL_Out) -> Kinetics/7(TireRL.Out)
  Forces/6(TireFR_Out) -> Kinetics/6(TireFR.Out)
  Forces/5(TireFL_Out) -> Kinetics/5(TireFL.Out)
  Forces/4(Car.Load) -> Kinetics/4(Car.Load)
  Forces/2(Car.Virtual) -> Kinetics/2(Car.Virtual)
  Kinematics/6(lSpring) -> Forces/6(lSpring)
  Kinematics/7(vDamp) -> Forces/7(vDamp)
  Forces/3(Car.Aero) -> Kinetics/3(Car.Aero)
  Forces/1(Sync_Out) -> Kinetics/1(Sync_In)
  Kinematics/5(TireRR_In) -> Forces/5(TireRR_In)
  Kinematics/4(TireRL_In) -> Forces/4(TireRL_In)
  Kinematics/3(TireFR_In) -> Forces/3(TireFR_In)
  Kinematics/2(TireFL_In) -> Forces/2(TireFL_In)
  Kinematics/1(Sync_Out) -> Forces/1(Sync_In)
  Kinematics/8(lStabi) -> Forces/8(lStabi)
  Forces/12(FBuf) -> Kinetics/12(FBuf)
  Kinematics/9(lBuf) -> Forces/9(lBuf)

== system TV_2018_HIL/CarMaker/IPG Vehicle3/PowerTrain ==
  note: When replacing the entire powertrain,
      | be sure to add '-disablepowertrain' to the command line arguments
      | in the CarMaker Model Configuration block.
  note: <Your model here>
  Sync_In : Inport
  Vhcl.Wheel.PT : Inport  Port=2
  VhclCtrl.PT : Inport  Port=3
  BusCreator1 : BusCreator  Inputs=42
  Demux1 : Demux  Outputs=42
  Electric Powertrain : Subsystem
  PowerTrain : S-Function  FunctionName=CM_Sfun  Parameters='PowerTrain'  SFunctionDeploymentMode=off  EnableBusSupport=off
  PowerTrainUpd : S-Function  FunctionName=CM_Sfun  Parameters='PowerTrainUpd'  SFunctionDeploymentMode=off  EnableBusSupport=off
  Saturation : Saturate  Commented=on  UpperLimit=2*pi*16000/60  LowerLimit=2*pi*100/60
  Terminator : Terminator
  Terminator1 : Terminator
  Sync_Out : Outport
  wires:
  BusCreator1/1 -> PowerTrainUpd/2
  Demux1/42 -> BusCreator1/42  "PT IF WRR Trq_BrakeReg_max"
  Demux1/41 -> BusCreator1/41  "PT IF WRR Trq_BrakeReg"
  Demux1/40 -> BusCreator1/40  "PT IF WRR Trq_Supp2WC"
  Demux1/38 -> BusCreator1/38  "PT IF WRR Trq_B2W"
  Demux1/37 -> BusCreator1/37  "PT IF WRR rotv"
  Demux1/36 -> BusCreator1/36  "PT IF WRR rot"
  Demux1/35 -> BusCreator1/35  "PT IF WRL Trq_BrakeReg_max"
  Demux1/34 -> BusCreator1/34  "PT IF WRL Trq_BrakeReg"
  Demux1/33 -> BusCreator1/33  "PT IF WRL Trq_Supp2WC"
  Demux1/31 -> BusCreator1/31  "PT IF WRL Trq_B2W"
  Demux1/30 -> BusCreator1/30  "PT IF WRL rotv"
  Demux1/29 -> BusCreator1/29  "PT IF WRL rot"
  Demux1/28 -> BusCreator1/28  "PT IF WFR Trq_BrakeReg_max"
  Demux1/27 -> BusCreator1/27  "PT IF WFR Trq_BrakeReg"
  Demux1/26 -> BusCreator1/26  "PT IF WFR Trq_Supp2WC"
  Demux1/24 -> BusCreator1/24  "PT IF WFR Trq_B2W"
  Demux1/23 -> BusCreator1/23  "PT IF WFR rotv"
  Demux1/22 -> BusCreator1/22  "PT IF WFR rot"
  Demux1/21 -> BusCreator1/21  "PT IF WFL Trq_BrakeReg_max"
  Demux1/20 -> BusCreator1/20  "PT IF WFL Trq_BrakeReg"
  Demux1/19 -> BusCreator1/19  "PT IF WFL Trq_Supp2WC"
  Demux1/17 -> BusCreator1/17  "PT IF WFL Trq_B2W"
  Demux1/16 -> BusCreator1/16  "PT IF WFL rotv"
  Demux1/15 -> BusCreator1/15  "PT IF WFL rot"
  Demux1/14 -> BusCreator1/14  "PT IF DL_iDiff_mean"
  Demux1/13 -> BusCreator1/13  "PT IF Trq_Supp2BdyEng y"
  Demux1/12 -> BusCreator1/12  "PT IF Trq_Supp2BdyEng x"
  Demux1/11 -> BusCreator1/11  "PT IF Trq_Supp2Bdy1B z"
  Demux1/10 -> BusCreator1/10  "PT IF Trq_Supp2Bdy1B y"
  Demux1/9 -> BusCreator1/9  "PT IF Trq_Supp2Bdy1B x"
  Demux1/8 -> BusCreator1/8  "PT IF Trq_Supp2Bdy1 z"
  Demux1/7 -> BusCreator1/7  "PT IF Trq_Supp2Bdy1 y"
  Demux1/6 -> BusCreator1/6  "PT IF Trq_Supp2Bdy1 x"
  Demux1/4 -> BusCreator1/4  "PT IF GearNo"
  Demux1/3 -> BusCreator1/3  "PT IF OperationError"
  Demux1/1 -> BusCreator1/1  "PT IF Ignition"
  Sync_In/1 -> PowerTrain/1
  PowerTrain/2 -> Demux1/1
  PowerTrainUpd/1 -> Sync_Out/1
  PowerTrain/1 -> PowerTrainUpd/1  "Sync"
  VhclCtrl.PT/1 -> PowerTrain/3
  Vhcl.Wheel.PT/1 -> PowerTrain/2
  Demux1/2 -> Terminator/1  "PT IF OperationState"
  Demux1/5 -> Terminator1/1  "PT IF Engine_rotv"
  Electric Powertrain/1(PT.OperationState1) -> BusCreator1/2
  Electric Powertrain/2(PT.Engine.rotv1) -> BusCreator1/5
  Electric Powertrain/3(T_FL) -> BusCreator1/18
  Electric Powertrain/4(T_FR) -> BusCreator1/25
  Electric Powertrain/5(T_RL) -> BusCreator1/32
  Electric Powertrain/6(T_RR) -> BusCreator1/39

== system TV_2018_HIL/CarMaker/Send sensor data and driver input to microcontroller /If Action Subsystem ==
  Action Port : ActionPort
  CAN Pack23 : canmsglib/CAN Pack  MsgList=(none)  MsgName=CAN Msg  MsgIDType=Standard (11-bit identifier)  MsgIdentifier=RESET_INVERTER  MsgLength=0  NSignals=0  StartBits=0  SignalSizes=0  ByteOrders=0  DataTypes=0  MultiplexTypes=0  MultiplexValues=0  Factors=0  Offsets=0  Minimums=0  Maximums=0  Remote=off
      settings: DataFormat=manually specified signals
  CAN Transmit23 : canlib/CAN Transmit  BlockHandle=3110.0001  DeviceMenu=(none)  Device=PEAK-System PCAN-PCI Express (PCAN_PCIBUS1)  ObjConstructor=canChannel('PEAK-System', 'PCAN_PCIBUS1')  EnablePeriodicTransmit=off  MessagePeriod=1.000
  wires:
  CAN Pack23/1 -> CAN Transmit23/1
